simulink model "Bahnplanung_lauffaehig_auf_Robotino"  (R2015b)
settings: Solver=ode3  StartTime=0.0  StopTime=inf  FixedStep=0.005  RelTol=1e-3
undefined symbols (not defined in the file or in its folder): Com1, none
libraries: xpcobsoletelib x4, xpcrtudplib x3, simulink x2, xpcseriallib x1, slrtlib x1
(part 1 of 2)
CloseFcn:
  | rtwprivate ssgencode ModelCloseRequest Robotino_Strecke_reall_2009
settings Model: SimulationMode=external  Creator=atlabor  LastModifiedBy=atlabor
settings SolverCC: EnableConcurrentExecution=on
settings DataIOCC: LimitDataPoints=off  SaveFormat=Array  SignalLoggingSaveFormat=ModelDataLogs
settings OptimizationCC: BlockReduction=off  OptimizeBlockIOStorage=off  BufferReuse=off  GlobalBufferReuse=off  ExpressionFolding=off  ExpressionDepthLimit=2147483647  LocalBlockOutputs=off  InitFltsAndDblsToZero=on
settings DebuggingCC: SaveWithParameterizedLinksMsg=none  UnderspecifiedInitializationDetection=Classic  MergeDetectMultiDrivingBlocksExec=none  SolverPrmCheckMsg=warning  FcnCallInpInsideContextMsg=UseLocalSettings  StateNameClashWarn=warning
settings HardwareCC: ProdBitPerPointer=32  ProdLargestAtomicFloat=None  ProdWordSize=32  ProdLongLongMode=on  ProdHWDeviceType=Generic->32-bit x86 compatible
settings SFSimCC: SimParseCustomCode=off
settings RTWCC: SystemTargetFile=slrt.tlc  TemplateMakefile=slrt_default_tmf  Description=Simulink Real-Time  RTWCompilerOptimization=on
settings SimulinkRealTimeCC: GeneratePreprocessorConditionals=Disable all
settings ConfigComp: CovModelRefEnable=Off  CovSFcnEnable=off

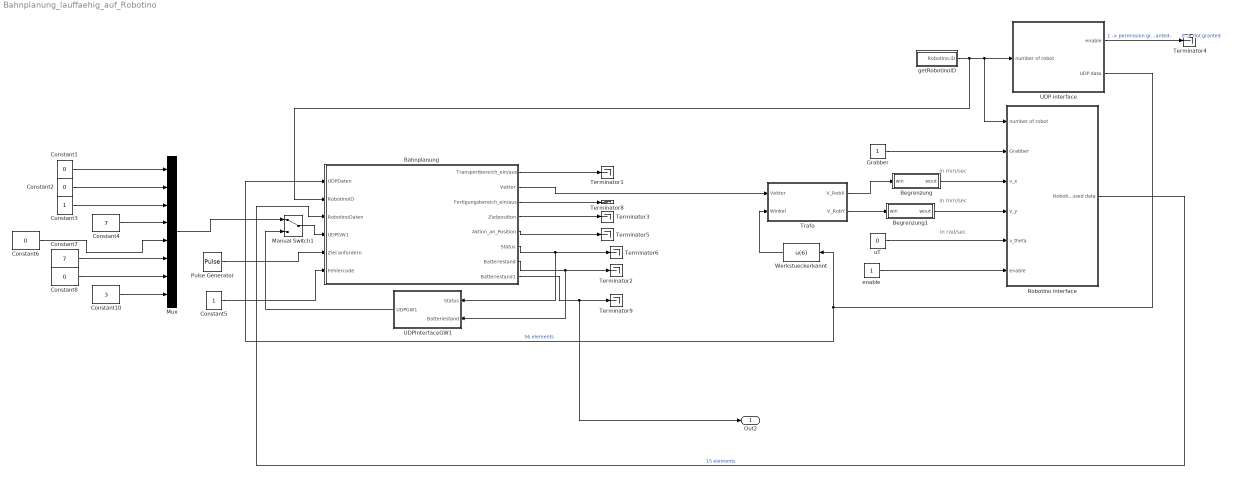
== system Bahnplanung_lauffaehig_auf_Robotino ==
  note: in rad/sec
  note: in mm/sec
  note: in mm/sec
  Bahnplanung : Subsystem
  Begrenzung : MATLAB Function  TreatAsAtomicUnit=on
  Begrenzung1 : MATLAB Function  TreatAsAtomicUnit=on
  Constant{1..2,6,8} (4 alike) : Constant  Value=0
  Constant10 : Constant  Value=3
  Constant3 : Constant
  Constant4 : Constant  Value=7
  Constant5 : Constant
  Constant7 : Constant  Value=7
  Grabber : Constant
  Manual Switch1 : ManualSwitch
  Mux : Mux  Inputs=8
  Pulse Generator : DiscretePulseGenerator  PulseType=Time based  Period=5  PulseWidth=50
  Robotino interface : Subsystem
  Terminator{1..6,8..9} (8 alike) : Terminator
  Trafo : MATLAB Function  TreatAsAtomicUnit=on
  UDP interface : Subsystem
  UDPInterfaceGW1 : Subsystem
  Werkstueckerkannt : Fcn  Expr=u(6)
  enable : Constant
  getRobotinoID : Subsystem
  uT : Constant  Value=0
  Out2 : Outport
  wires:
  Robotino interface/1(Robotino processed data) -> Bahnplanung/3(RobotinoDaten)  "15 elements"
  UDP interface/2(UDP data) -> Bahnplanung/1(UDPDaten), Werkstueckerkannt/1  "56 elements"
  uT/1 -> Robotino interface/5(v_theta)
  UDP interface/1(enable) -> Terminator4/1  "1 -> permission granted;        0 -> not granted"
  enable/1 -> Robotino interface/6(enable)
  getRobotinoID/1(Robotino.ID) -> Bahnplanung/2(RobotinoID), Robotino interface/1(number of robot), UDP interface/1(number of robot)
  Grabber/1 -> Robotino interface/2(Grabber)
  Constant5/1 -> Bahnplanung/6(Fehlercode)
  Pulse Generator/1 -> Bahnplanung/5(Ziel anfordern)
  Bahnplanung/1(Transportbereich_ein/aus) -> Terminator1/1
  Bahnplanung/4(Zielposition) -> Terminator3/1
  Bahnplanung/5(Aktion_an_Position) -> Terminator5/1
  Bahnplanung/6(Status) -> Terminator6/1, UDPInterfaceGW1/1(Status)
  Bahnplanung/7(Batteriestand) -> Terminator2/1, UDPInterfaceGW1/2(Batteriestand)
  Bahnplanung/3(Fertigungsbereich_ein/aus) -> Terminator8/1
  Constant1/1 -> Mux/1
  Constant2/1 -> Mux/2
  Constant3/1 -> Mux/3
  Constant6/1 -> Mux/5
  Constant7/1 -> Mux/6
  Constant8/1 -> Mux/7
  Constant10/1 -> Mux/8
  Begrenzung/1(wout) -> Robotino interface/3(v_x)
  Trafo/2(V_RobY) -> Begrenzung1/1(win)
  Werkstueckerkannt/1 -> Trafo/2(Winkel)
  Trafo/1(V_RobX) -> Begrenzung/1(win)
  Begrenzung1/1(wout) -> Robotino interface/4(v_y)
  Constant4/1 -> Mux/4
  Manual Switch1/1 -> Bahnplanung/4(UDPGW1)
  Mux/1 -> Manual Switch1/1
  UDPInterfaceGW1/1(UDPGW1) -> Manual Switch1/2
  Bahnplanung/8(Batteriestand1) -> Out2/1, Terminator9/1
  Bahnplanung/2(Vektor) -> Trafo/1(Vektor)

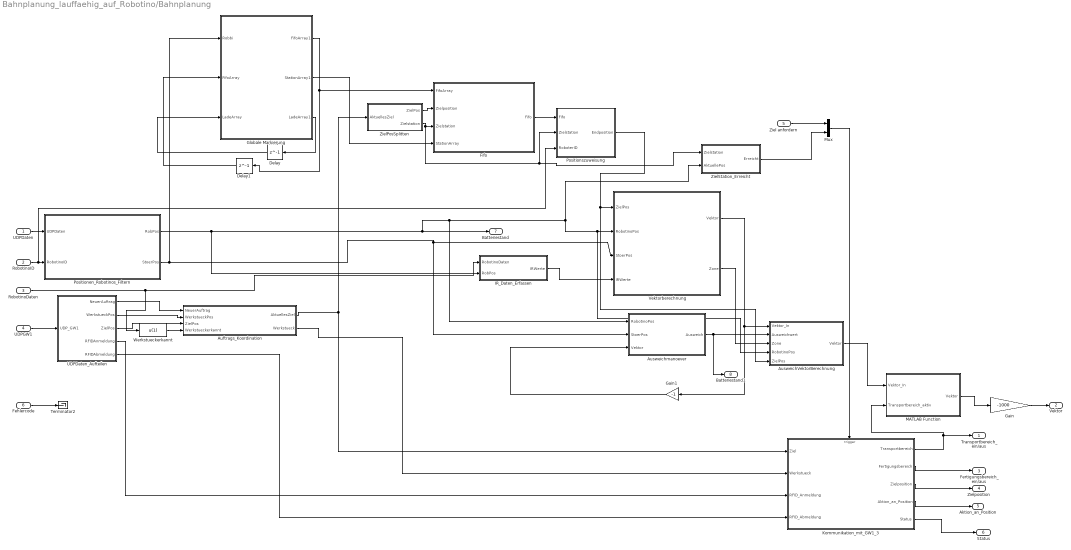
== system Bahnplanung_lauffaehig_auf_Robotino/Bahnplanung ==
  UDPDaten : Inport  PortDimensions=56
  RobotinoID : Inport  Port=2
  RobotinoDaten : Inport  Port=3
  UDPGW1 : Inport  Port=4
  Ziel anfordern : Inport  Port=5
  Fehlercode : Inport  Port=6
  Auftrags_Koordination : Stateflow chart  TreatAsAtomicUnit=on
  AusweichVektorBerechnung : MATLAB Function  TreatAsAtomicUnit=on
  Ausweichmanoever : MATLAB Function  TreatAsAtomicUnit=on
  Delay : Delay  DelayLength=1
  Delay1 : Delay  DelayLength=1
  Fifo : Stateflow chart  TreatAsAtomicUnit=on
  Gain : Gain  Gain=-1000
  Gain1 : Gain  Gain=-1
  Globale Markierung : MATLAB Function  TreatAsAtomicUnit=on
  IR_Daten_Erfassen : MATLAB Function  TreatAsAtomicUnit=on
  Kommunikation_mit_GW1_3 : Stateflow chart  TreatAsAtomicUnit=on
  MATLAB Function : MATLAB Function  TreatAsAtomicUnit=on
  Mux : Mux  Inputs=2
  Positionen_Robotinos_Filtern : MATLAB Function  TreatAsAtomicUnit=on
  Positionszuweisung : MATLAB Function  TreatAsAtomicUnit=on
  Terminator2 : Terminator
  UDPDaten_Aufteilen : Subsystem
  Vektorberechnung : MATLAB Function  TreatAsAtomicUnit=on
  Werkstueckerkannt : Fcn  Expr=u(1)
  ZielPosSplitten : MATLAB Function  TreatAsAtomicUnit=on
  ZielStation_Erreicht : MATLAB Function  TreatAsAtomicUnit=on
  Transportbereich_ein/aus : Outport
  Vektor : Outport  Port=2  OutDataTypeStr=double  PortDimensions=[1 2]
  Fertigungsbereich_ein/aus : Outport  Port=3
  Zielposition : Outport  Port=4
  Aktion_an_Position : Outport  Port=5
  Status : Outport  Port=6
  Batteriestand : Outport  Port=7
  Batteriestand1 : Outport  Port=8
  wires:
  RobotinoID/1 -> Positionszuweisung/3(RoboterID), Positionen_Robotinos_Filtern/2(RobotinoID)
  UDPDaten/1 -> Positionen_Robotinos_Filtern/1(UDPDaten)
  Positionen_Robotinos_Filtern/2(StoerPos) -> Ausweichmanoever/2(StoerPos), Vektorberechnung/3(StoerPos), Globale Markierung/1(Robbi)
  Globale Markierung/2(StationArray1) -> Fifo/4(StationArray)
  RobotinoDaten/1 -> IR_Daten_Erfassen/1(RobotinoDaten), Werkstueckerkannt/1
  Kommunikation_mit_GW1_3/3(Zielposition) -> Zielposition/1
  Kommunikation_mit_GW1_3/4(Aktion_an_Position) -> Aktion_an_Position/1
  Kommunikation_mit_GW1_3/2(Fertigungsbereich) -> Fertigungsbereich_ein/aus/1
  Kommunikation_mit_GW1_3/1(Transportbereich) -> Transportbereich_ein/aus/1, MATLAB Function/2(Transportbereich_aktiv)
  UDPGW1/1 -> UDPDaten_Aufteilen/1(UDP_GW1)
  UDPDaten_Aufteilen/4(RFIDAnmeldung) -> Kommunikation_mit_GW1_3/3(RFID_Anmeldung)
  UDPDaten_Aufteilen/5(RFIDAbmeldung) -> Kommunikation_mit_GW1_3/4(RFID_Abmeldung)
  UDPDaten_Aufteilen/2(WerkstueckPos) -> Auftrags_Koordination/2(WerkstueckPos)
  UDPDaten_Aufteilen/3(ZielPos) -> Auftrags_Koordination/3(ZielPos)
  Auftrags_Koordination/1(AktuellesZiel) -> ZielPosSplitten/1(AktuellesZiel), Kommunikation_mit_GW1_3/1(Ziel)
  ZielPosSplitten/1(ZielPos) -> Fifo/2(Zielposition)
  ZielPosSplitten/2(Zielstation) -> ZielStation_Erreicht/1(Zielstation), Positionszuweisung/2(Zielstation), Fifo/3(Zielstation)
  Fehlercode/1 -> Terminator2/1
  UDPDaten_Aufteilen/1(NeuerAuftrag) -> Auftrags_Koordination/1(NeuerAuftrag)
  Auftrags_Koordination/2(Werkstueck) -> Kommunikation_mit_GW1_3/2(Werkstueck)
  Werkstueckerkannt/1 -> Auftrags_Koordination/4(Werkstueckerkannt)
  Globale Markierung/1(FifoArray1) -> Delay1/1, Fifo/1(FifoArray)
  Delay1/1 -> Globale Markierung/2(FifoArray)
  Fifo/1(Fifo) -> Positionszuweisung/1(Fifo)
  Positionszuweisung/1(Endposition) -> AusweichVektorBerechnung/5(ZielPos), Vektorberechnung/1(ZielPos)
  Kommunikation_mit_GW1_3/5(Status) -> Status/1
  Globale Markierung/3(LadeArray1) -> Delay/1
  Delay/1 -> Globale Markierung/3(LadeArray)
  Mux/1 -> Kommunikation_mit_GW1_3/Trigger
  Ziel anfordern/1 -> Mux/1
  ZielStation_Erreicht/1(Erreicht) -> Mux/2
  MATLAB Function/1(Vektor) -> Gain/1
  Ausweichmanoever/1(Ausweich) -> Batteriestand1/1, AusweichVektorBerechnung/2(Ausweichwert)
  Gain/1 -> Vektor/1
  Vektorberechnung/1(Vektor) -> AusweichVektorBerechnung/1(Vektor_In), Gain1/1
  Gain1/1 -> Ausweichmanoever/3(Vektor)
  Positionen_Robotinos_Filtern/1(RobPos) -> IR_Daten_Erfassen/2(RobPos), Batteriestand/1, Ausweichmanoever/1(RobotinoPos), ZielStation_Erreicht/2(AktuellePos), AusweichVektorBerechnung/4(RobotinoPos), Vektorberechnung/2(RobotinoPos)
  IR_Daten_Erfassen/1(IRWerte) -> Vektorberechnung/4(IRWerte)
  AusweichVektorBerechnung/1(Vektor) -> MATLAB Function/1(Vektor_In)
  Vektorberechnung/2(Zone) -> AusweichVektorBerechnung/3(Zone)

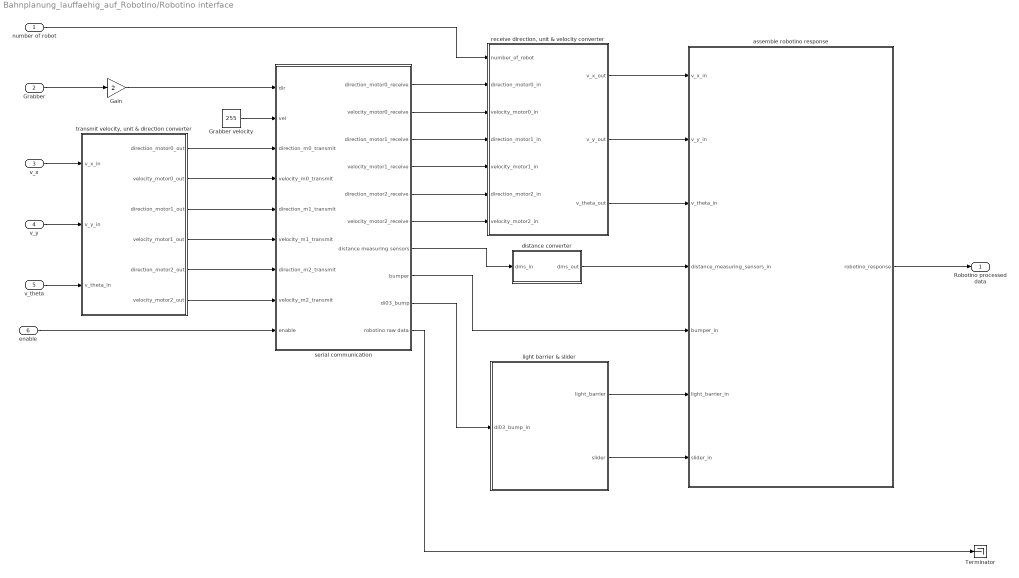
== system Bahnplanung_lauffaehig_auf_Robotino/Robotino interface ==
  number of robot : Inport
  Grabber : Inport  Port=2
  v_x : Inport  Port=3
  v_y : Inport  Port=4
  v_theta : Inport  Port=5
  enable : Inport  Port=6
  Gain : Gain  Gain=2
  Grabber velocity : Constant  Value=255
  Terminator : Terminator
  assemble robotino response : MATLAB Function  TreatAsAtomicUnit=on
  distance converter : MATLAB Function  TreatAsAtomicUnit=on
  light barrier & slider : MATLAB Function  TreatAsAtomicUnit=on
  "receive direction, unit & velocity converter" : MATLAB Function  TreatAsAtomicUnit=on
  serial communication : Subsystem
  "transmit velocity, unit & direction converter" : MATLAB Function  TreatAsAtomicUnit=on
  Robotino processed data : Outport
  wires:
  "transmit velocity, unit & direction converter"/1(direction_motor0_out) -> serial communication/3(direction_m0_transmit)
  "transmit velocity, unit & direction converter"/2(velocity_motor0_out) -> serial communication/4(velocity_m0_transmit)
  "transmit velocity, unit & direction converter"/3(direction_motor1_out) -> serial communication/5(direction_m1_transmit)
  "transmit velocity, unit & direction converter"/4(velocity_motor1_out) -> serial communication/6(velocity_m1_transmit)
  "transmit velocity, unit & direction converter"/5(direction_motor2_out) -> serial communication/7(direction_m2_transmit)
  "transmit velocity, unit & direction converter"/6(velocity_motor2_out) -> serial communication/8(velocity_m2_transmit)
  v_x/1 -> "transmit velocity, unit & direction converter"/1(v_x_in)
  v_y/1 -> "transmit velocity, unit & direction converter"/2(v_y_in)
  v_theta/1 -> "transmit velocity, unit & direction converter"/3(v_theta_in)
  "receive direction, unit & velocity converter"/2(v_y_out) -> assemble robotino response/2(v_y_in)
  enable/1 -> serial communication/9(enable)
  serial communication/1(direction_motor0_receive) -> "receive direction, unit & velocity converter"/2(direction_motor0_in)
  serial communication/7(distance measuring sensors) -> distance converter/1(dms_in)
  serial communication/10(robotino raw data) -> Terminator/1
  serial communication/9(di03_bump) -> light barrier & slider/1(di03_bump_in)
  "receive direction, unit & velocity converter"/1(v_x_out) -> assemble robotino response/1(v_x_in)
  "receive direction, unit & velocity converter"/3(v_theta_out) -> assemble robotino response/3(v_theta_in)
  assemble robotino response/1(robotino_response) -> Robotino processed data/1
  Grabber/1 -> Gain/1
  Gain/1 -> serial communication/1(dir)
  distance converter/1(dms_out) -> assemble robotino response/4(distance_measuring_sensors_in)
  light barrier & slider/2(slider) -> assemble robotino response/7(slider_in)
  light barrier & slider/1(light_barrier) -> assemble robotino response/6(light_barrier_in)
  serial communication/8(bumper) -> assemble robotino response/5(bumper_in)
  serial communication/2(velocity_motor0_receive) -> "receive direction, unit & velocity converter"/3(velocity_motor0_in)
  serial communication/3(direction_motor1_receive) -> "receive direction, unit & velocity converter"/4(direction_motor1_in)
  serial communication/4(velocity_motor1_receive) -> "receive direction, unit & velocity converter"/5(velocity_motor1_in)
  serial communication/5(direction_motor2_receive) -> "receive direction, unit & velocity converter"/6(direction_motor2_in)
  serial communication/6(velocity_motor2_receive) -> "receive direction, unit & velocity converter"/7(velocity_motor2_in)
  Grabber velocity/1 -> serial communication/2(vel)
  number of robot/1 -> "receive direction, unit & velocity converter"/1(number_of_robot)

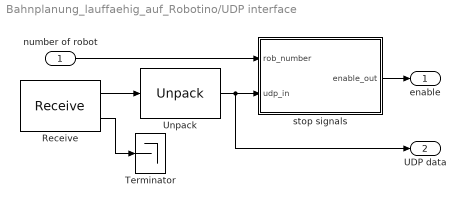
== system Bahnplanung_lauffaehig_auf_Robotino/UDP interface ==
  number of robot : Inport
  Receive : xpcrtudplib/Legacy UDP/Receive   ipAddress=0.0.0.0  ipPort=25000  width=448  vblLen=off  sampletime=-1
  Terminator : Terminator
  Unpack : xpcobsoletelib/Utilities/Unpack   dimensions={[56]}  datatypes={'double'}  byteAlign=1
  stop signals : MATLAB Function  TreatAsAtomicUnit=on
  enable : Outport
  UDP data : Outport  Port=2
  wires:
  Unpack/1 -> stop signals/2(udp_in), UDP data/1
  Receive/1 -> Unpack/1
  Receive/2 -> Terminator/1
  stop signals/1(enable_out) -> enable/1
  number of robot/1 -> stop signals/1(rob_number)

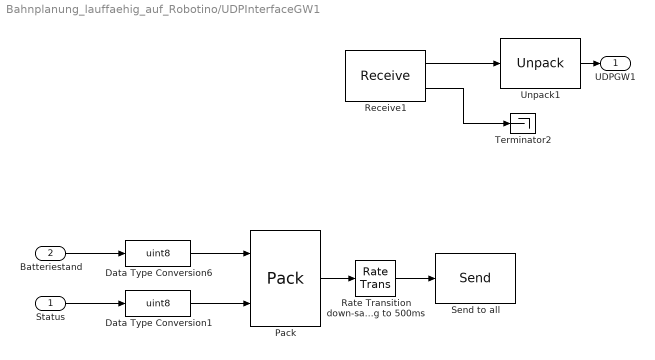
== system Bahnplanung_lauffaehig_auf_Robotino/UDPInterfaceGW1 ==
  Status : Inport
  Batteriestand : Inport  Port=2
  Data Type Conversion1 : DataTypeConversion  OutDataTypeStr=uint8
  Data Type Conversion6 : DataTypeConversion  OutDataTypeStr=uint8
  Pack : xpcobsoletelib/Utilities/Pack   datatypes={'int16','int16'}  byteAlign=1
  Rate Transition down-sampling to 500ms : RateTransition  OutPortSampleTime=0.5
  Receive1 : xpcrtudplib/Legacy UDP/Receive   ipAddress=0.0.0.0  ipPort=20000  width=448  vblLen=off  sampletime=-1
  Send to all : xpcrtudplib/Legacy UDP/Send   ipAddress=255.255.255.255  ipPort=20000  localPort=-1  vblLen=off  sampletime=-1
  Terminator2 : Terminator
  Unpack1 : xpcobsoletelib/Utilities/Unpack   dimensions={[8]}  datatypes={'int8'}  byteAlign=1
  UDPGW1 : Outport
  wires:
  Receive1/2 -> Terminator2/1
  Unpack1/1 -> UDPGW1/1
  Receive1/1 -> Unpack1/1
  Pack/1 -> Rate Transition down-sampling to 500ms/1
  Rate Transition down-sampling to 500ms/1 -> Send to all/1
  Data Type Conversion1/1 -> Pack/2
  Data Type Conversion6/1 -> Pack/1
  Batteriestand/1 -> Data Type Conversion6/1
  Status/1 -> Data Type Conversion1/1

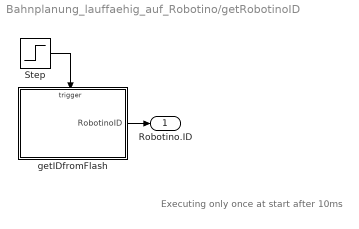
== system Bahnplanung_lauffaehig_auf_Robotino/getRobotinoID ==
  note: Executing only once at start after 10ms
  Step : Step  Time=0.01  SampleTime=0
  getIDfromFlash : Subsystem
  Robotino.ID : Outport
  wires:
  Step/1 -> getIDfromFlash/Trigger
  getIDfromFlash/1(RobotinoID) -> Robotino.ID/1

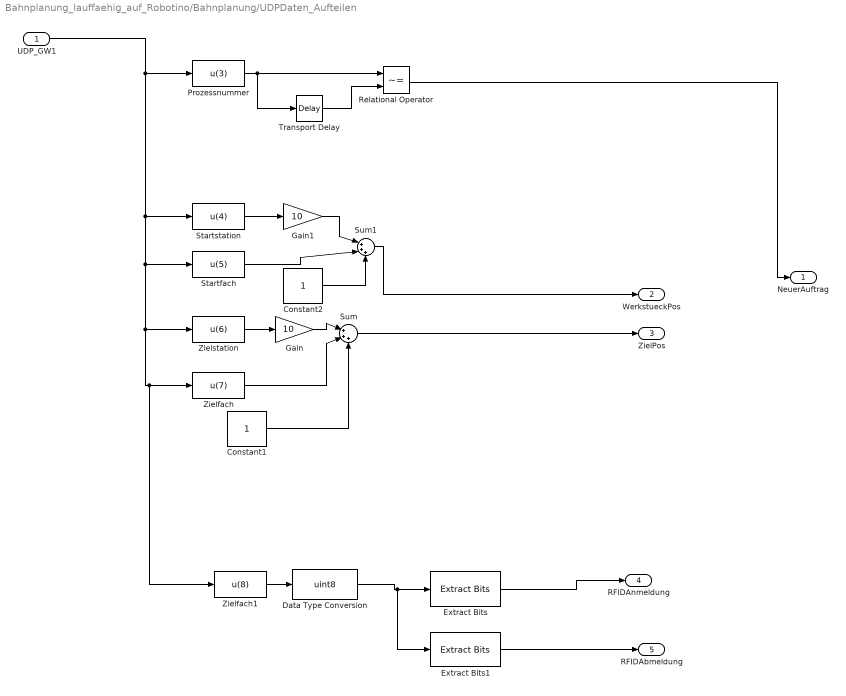
== system Bahnplanung_lauffaehig_auf_Robotino/Bahnplanung/UDPDaten_Aufteilen ==
  UDP_GW1 : Inport
  Constant1 : Constant
  Constant2 : Constant
  Data Type Conversion : DataTypeConversion  OutDataTypeStr=uint8
  Extract Bits : simulink/Logic and Bit Operations/Extract Bits  bitsToExtract=Range of bits  numBits=8  bitIdxRange=[0]  outScalingMode=Treat bit field as an integer
  Extract Bits1 : simulink/Logic and Bit Operations/Extract Bits  bitsToExtract=Range of bits  numBits=8  bitIdxRange=[1]  outScalingMode=Treat bit field as an integer
  Gain : Gain  Gain=10
  Gain1 : Gain  Gain=10
  Prozessnummer : Fcn  Expr=u(3)
  Relational Operator : RelationalOperator  Operator=~=  OutDataTypeStr=boolean
  Startfach : Fcn  Expr=u(5)
  Startstation : Fcn  Expr=u(4)
  Sum : Sum  Inputs=|+++
  Sum1 : Sum  Inputs=|+++
  Transport Delay : TransportDelay
  Zielfach : Fcn  Expr=u(7)
  Zielfach1 : Fcn  Expr=u(8)
  Zielstation : Fcn  Expr=u(6)
  NeuerAuftrag : Outport
  WerkstueckPos : Outport  Port=2
  ZielPos : Outport  Port=3
  RFIDAnmeldung : Outport  Port=4
  RFIDAbmeldung : Outport  Port=5
  wires:
  Zielfach/1 -> Sum/2
  Gain/1 -> Sum/1
  Zielstation/1 -> Gain/1
  UDP_GW1/1 -> Prozessnummer/1, Zielfach1/1, Zielfach/1, Zielstation/1, Startfach/1, Startstation/1
  Sum1/1 -> WerkstueckPos/1
  Startfach/1 -> Sum1/2
  Gain1/1 -> Sum1/1
  Constant2/1 -> Sum1/3
  Startstation/1 -> Gain1/1
  Constant1/1 -> Sum/3
  Sum/1 -> ZielPos/1
  Relational Operator/1 -> NeuerAuftrag/1
  Zielfach1/1 -> Data Type Conversion/1
  Data Type Conversion/1 -> Extract Bits1/1, Extract Bits/1
  Prozessnummer/1 -> Transport Delay/1, Relational Operator/1
  Transport Delay/1 -> Relational Operator/2
  Extract Bits1/1 -> RFIDAbmeldung/1
  Extract Bits/1 -> RFIDAnmeldung/1

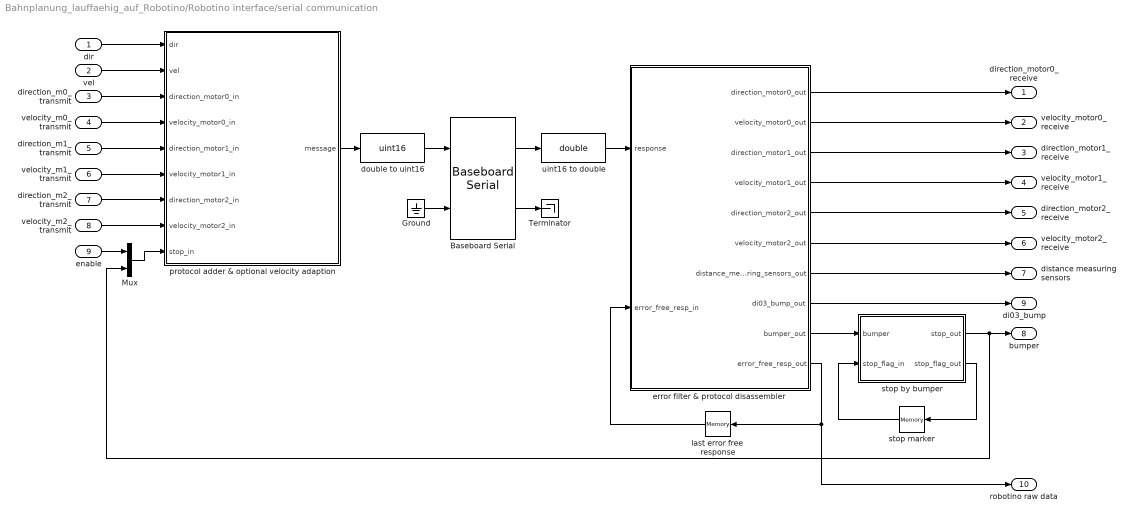
== system Bahnplanung_lauffaehig_auf_Robotino/Robotino interface/serial communication ==
  dir : Inport
  vel : Inport  Port=2
  direction_m0_transmit : Inport  Port=3
  velocity_m0_transmit : Inport  Port=4
  direction_m1_transmit : Inport  Port=5
  velocity_m1_transmit : Inport  Port=6
  direction_m2_transmit : Inport  Port=7
  velocity_m2_transmit : Inport  Port=8
  enable : Inport  Port=9
  Baseboard Serial : xpcseriallib/Mainboard/Baseboard Serial  group=Transmit Setup  port=2  irqnum=4  saddr1=0x3f8  saddr2=0x3e8  config=Com1/none  baud1=115200  parity1=None  ndata1=8  nstop1=1  fifomode1=16 deep  rlevel1=almost full  automode1=off  xmtfifosize1=10240  xmtdatatype1=count+16 bit uint  rcvfifosize1=10240  rcvmaxread1=101  rcvminread1=1  rcvusedelim1=on  rcvdelim1=99  rcvdatatype1=count+16 bit uint  rcvsampletime1=-1  baud2=115200  parity2=None  ndata2=8  nstop2=1  fifomode2=16 deep  rlevel2=almost full  automode2=off  xmtfifosize2=10240  xmtdatatype2=count+16 bit uint  rcvfifosize2=10240  rcvmaxread2=101  rcvminread2=1  rcvusedelim2=on  rcvdelim2=99  rcvdatatype2=count+16 bit uint  rcvsampletime2=-1
      link override FIFO read 1: maxsize=101  minsize=1  usedelimiter=on  delimiter=99  outputtype=count+16 bit uint  sampletime=dt / 2
      link override FIFO read 2: maxsize=101  minsize=1  usedelimiter=on  delimiter=99  outputtype=count+16 bit uint  sampletime=dt / 2
      link override FIFO write 1: size=1024  inputtype=count+16 bit uint  sampletime=-1  id=XMT channel 1, IRQ 4
      link override FIFO write 2: size=1024  inputtype=8 bit uint null terminated  id=XMT channel 2, IRQ 4
      link override Setup1: baud=115200  width=8  nstop=1  parity=None  fmode=16 deep  rlevel=half full  ctsmode=off
      link override Setup2: baud=4800  width=8  nstop=1  parity=None  fmode=16 deep  rlevel=half full  ctsmode=off
  Ground : Ground
  Mux : Mux  Inputs=2
  Terminator : Terminator
  double to uint16 : DataTypeConversion  OutDataTypeStr=uint16  RndMeth=Nearest
  error filter & protocol disassembler : MATLAB Function  TreatAsAtomicUnit=on
  last error free response : Memory  X0=[zeros(1,102)]
  protocol adder & optional velocity adaption : MATLAB Function  TreatAsAtomicUnit=on
  stop by bumper : MATLAB Function  TreatAsAtomicUnit=on
  stop marker : Memory  X0=[zeros(1,3)]
  uint16 to double : DataTypeConversion  OutDataTypeStr=double  RndMeth=Nearest
  direction_motor0_receive : Outport
  velocity_motor0_receive : Outport  Port=2
  direction_motor1_receive : Outport  Port=3
  velocity_motor1_receive : Outport  Port=4
  direction_motor2_receive : Outport  Port=5
  velocity_motor2_receive : Outport  Port=6
  distance measuring sensors : Outport  Port=7
  bumper : Outport  Port=8
  di03_bump : Outport  Port=9
  robotino raw data : Outport  Port=10
  wires:
  Ground/1 -> Baseboard Serial/2
  Baseboard Serial/2 -> Terminator/1
  double to uint16/1 -> Baseboard Serial/1
  protocol adder & optional velocity adaption/1(message) -> double to uint16/1
  stop marker/1 -> stop by bumper/2(stop_flag_in)
  stop by bumper/2(stop_flag_out) -> stop marker/1
  last error free response/1 -> error filter & protocol disassembler/2(error_free_resp_in)
  error filter & protocol disassembler/10(error_free_resp_out) -> last error free response/1, robotino raw data/1
  error filter & protocol disassembler/1(direction_motor0_out) -> direction_motor0_receive/1
  error filter & protocol disassembler/2(velocity_motor0_out) -> velocity_motor0_receive/1
  error filter & protocol disassembler/3(direction_motor1_out) -> direction_motor1_receive/1
  error filter & protocol disassembler/4(velocity_motor1_out) -> velocity_motor1_receive/1
  direction_m0_transmit/1 -> protocol adder & optional velocity adaption/3(direction_motor0_in)
  error filter & protocol disassembler/5(direction_motor2_out) -> direction_motor2_receive/1
  velocity_m0_transmit/1 -> protocol adder & optional velocity adaption/4(velocity_motor0_in)
  error filter & protocol disassembler/6(velocity_motor2_out) -> velocity_motor2_receive/1
  direction_m1_transmit/1 -> protocol adder & optional velocity adaption/5(direction_motor1_in)
  velocity_m1_transmit/1 -> protocol adder & optional velocity adaption/6(velocity_motor1_in)
  direction_m2_transmit/1 -> protocol adder & optional velocity adaption/7(direction_motor2_in)
  velocity_m2_transmit/1 -> protocol adder & optional velocity adaption/8(velocity_motor2_in)
  error filter & protocol disassembler/9(bumper_out) -> stop by bumper/1(bumper)
  stop by bumper/1(stop_out) -> bumper/1, Mux/2
  error filter & protocol disassembler/7(distance_measuring_sensors_out) -> distance measuring sensors/1
  Baseboard Serial/1 -> uint16 to double/1
  uint16 to double/1 -> error filter & protocol disassembler/1(response)
  enable/1 -> Mux/1
  dir/1 -> protocol adder & optional velocity adaption/1(dir)
  vel/1 -> protocol adder & optional velocity adaption/2(vel)
  Mux/1 -> protocol adder & optional velocity adaption/9(stop_in)
  error filter & protocol disassembler/8(di03_bump_out) -> di03_bump/1

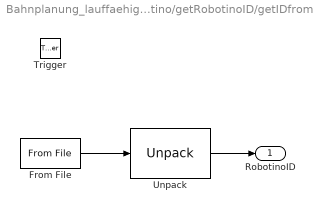
== system Bahnplanung_lauffaehig_auf_Robotino/getRobotinoID/getIDfromFlash ==
  Trigger : TriggerPort
  From File : slrtlib/Target Management/From File   filename='robotino.id'  dataSize=8  bufSize=2000  readSize=512  EOFOption=Seek to beginning  sampTime=-1  show2ports=off
  Unpack : xpcobsoletelib/Utilities/Unpack   dimensions={[1]}  datatypes={'double'}  byteAlign=1
  RobotinoID : Outport
  wires:
  From File/1 -> Unpack/1
  Unpack/1 -> RobotinoID/1

== matlab function Bahnplanung_lauffaehig_auf_Robotino/Robotino interface/transmit velocity, unit & direction converter ==
  settings: sampleTime=2*dtpc
  data: direction_motor0_out output; velocity_motor0_out output; direction_motor1_out output; velocity_motor1_out output; direction_motor2_out output; velocity_motor2_out output; v_x_in input; v_y_in input; v_theta_in input
%%%%%%%%%%%%%%%%%%%%%%%%%%%%%%%%%%%%%%%%%%%%%%%%%%%%%%%%%%%%%%%%%%%%%%%%%%%
% conversion from positive and/or negative longitudinal, lateral and      %
% rotational velocities (in milimeters per second) to three separate      %
% positive motor velocities (resolution: 1Byte) and their rotation        %
% direction                                                               %
%                                                                         %
% inputs:  v_x_in (longitudinal velocity in milimeters per second),       %
%          v_y_in (lateral velocity in milimeters per second),            %
%          v_theta_in (rotational velocity in milimeters per second)      %
% outputs: direction_motor0_out (rotating direction of motor0             %
%          (0 := counter-clockwise; 2 := clockwise)),                     %
%          velocity_motor0_out (from 0 to 255),                           %
%          direction_motor1_out (rotating direction of motor1             %
%          (0 := counter-clockwise; 2 := clockwise)),                     %
%          velocity_motor1_out (from 0 to 255),                           %
%          direction_motor2_out (rotating direction of motor2             %
%          (0 := counter-clockwise; 2 := clockwise)),                     %
%          velocity_motor2_out (from 0 to 255)                            %
%%%%%%%%%%%%%%%%%%%%%%%%%%%%%%%%%%%%%%%%%%%%%%%%%%%%%%%%%%%%%%%%%%%%%%%%%%%
function [direction_motor0_out, velocity_motor0_out, ...
          direction_motor1_out, velocity_motor1_out, ...
          direction_motor2_out, velocity_motor2_out] ...
                                          = fcn(v_x_in, v_y_in, v_theta_in)
%%%%%%%%%%%%%%%%%%%%%%%%%%%%%%%%%%%%%%%%%%%%%%%%%%%%%%%%%%%%%%%%%%%%%%
% conversion from longitudinal, lateral & rotational velocity to the %
% three separate motor velocities                                    %
%%%%%%%%%%%%%%%%%%%%%%%%%%%%%%%%%%%%%%%%%%%%%%%%%%%%%%%%%%%%%%%%%%%%%%
v0 = (-v_x_in * cosd(30)) + ( v_y_in * cosd(60)) + (v_theta_in * 135);
v1 =                      + (-v_y_in)            + (v_theta_in * 135);
v2 = ( v_x_in * cosd(30)) + ( v_y_in * cosd(60)) + (v_theta_in * 135);

%%%%%%%%%%%%%%%%%%%%%%%%%%%%%%%%%%%%%%%%%%%%%%%%%%%%%%%%%%%%%%%%%%%%%
% conversion of the separate motor velocities from millimeters to a %
% value between -255 and 255                                        %
%%%%%%%%%%%%%%%%%%%%%%%%%%%%%%%%%%%%%%%%%%%%%%%%%%%%%%%%%%%%%%%%%%%%%
f = 1 / 7.02;
v0 = v0 * f;
v1 = v1 * f;
v2 = v2 * f;

%%%%%%%%%%%%%%%%%%%%%%%%%%%%%%%%%%%%%%%%%%%%%%%%%%%%%%%%%%%%%%%%%%%%
% division of motor velocities into absolute velocity and rotating %
% direction                                                        %
%%%%%%%%%%%%%%%%%%%%%%%%%%%%%%%%%%%%%%%%%%%%%%%%%%%%%%%%%%%%%%%%%%%%
if v0 < 0
    direction_motor0_out =  0;
    velocity_motor0_out  = -v0;
else
    direction_motor0_out = 2;
    velocity_motor0_out  = v0;
end

if v1 < 0
    direction_motor1_out =  0;
    velocity_motor1_out  = -v1;
else
    direction_motor1_out = 2;
    velocity_motor1_out  = v1;
end

if v2 < 0
    direction_motor2_out =  0;
    velocity_motor2_out  = -v2;
else
    direction_motor2_out = 2;
    velocity_motor2_out  = v2;
end

== matlab function Bahnplanung_lauffaehig_auf_Robotino/Robotino interface/serial communication/protocol adder & optional velocity adaption ==
  settings: sampleTime=2*dtpc
  data: dir input; vel input; direction_motor0_in input; velocity_motor0_in input; direction_motor1_in input; velocity_motor1_in input; direction_motor2_in input; velocity_motor2_in input; stop_in input; message output
%%%%%%%%%%%%%%%%%%%%%%%%%%%%%%%%%%%%%%%%%%%%%%%%%%%%%%%%%%%%%%%%%%%%%%%%%%%
% parameterising the 'PC104 to I/O-Board message' for serial line         %
% communication with control commands for the robotino motors             %
%                                                                         %
% optional: velocity adaption as soon as at least one motor is near the   %
%           speed limit                                                   %
%                                                                         %
% inputs: rotating directions and velocities of the three motors          %
% output: vector containing the 'PC104 to I/O-Board message' for serial   %
%         line communication                                              %
%%%%%%%%%%%%%%%%%%%%%%%%%%%%%%%%%%%%%%%%%%%%%%%%%%%%%%%%%%%%%%%%%%%%%%%%%%%
function message = fcn(dir, vel, direction_motor0_in, velocity_motor0_in, ...
                       direction_motor1_in, velocity_motor1_in, ...
                       direction_motor2_in, velocity_motor2_in, stop_in)
%%%%%%%%%%%%%%%%%%%%%%%%%%%%%%
% optional velocity adaption %
%%%%%%%%%%%%%%%%%%%%%%%%%%%%%%
vmax = 175;                                               % v_motor_dez_max

if velocity_motor0_in > vmax
    velocity_motor0_tf = velocity_motor0_in;
    
    velocity_motor0_in = vmax;
    velocity_motor1_in = vmax * velocity_motor1_in / velocity_motor0_tf;
    velocity_motor2_in = vmax * velocity_motor2_in / velocity_motor0_tf;
end

if velocity_motor1_in > vmax
    velocity_motor1_tf = velocity_motor1_in;
    
    velocity_motor0_in = vmax * velocity_motor0_in / velocity_motor1_tf;
    velocity_motor1_in = vmax;
    velocity_motor2_in = vmax * velocity_motor2_in / velocity_motor1_tf;
end

if velocity_motor2_in > vmax
    velocity_motor2_tf = velocity_motor2_in;
    
    velocity_motor0_in = vmax * velocity_motor0_in / velocity_motor2_tf;
    velocity_motor1_in = vmax * velocity_motor1_in / velocity_motor2_tf;
    velocity_motor2_in = vmax;
end
%%%%%%%%%%%%%%%%%%%%%%%%%%%%%%%%%%%%%%%%%%%%%%%%%%%%%%%%%%%%%%%%%%%%%%
% vector containing the 'PC104 to I/O-Board message' for serial line %
% communication                                                      %
%%%%%%%%%%%%%%%%%%%%%%%%%%%%%%%%%%%%%%%%%%%%%%%%%%%%%%%%%%%%%%%%%%%%%%
message = [47, abs('REC'), 5, min(stop_in), direction_motor0_in, ...
           velocity_motor0_in, zeros(1, 4), 255, 255, 255, ...
           min(stop_in), direction_motor1_in, velocity_motor1_in, ...
           zeros(1, 4), 255, 255, 255, min(stop_in), ...
           direction_motor2_in, velocity_motor2_in, zeros(1, 4), 255, ...
           255, 255, 1, dir, vel, zeros(1, 4), 255, 255, 255, abs('rec')].';

== matlab function Bahnplanung_lauffaehig_auf_Robotino/UDP interface/stop signals ==
  data: rob_number input; udp_in input; enable_out output
%%%%%%%%%%%%%%%%%%%%%%%%%%%%%%%%%%%%%%%%%%%%%%%%%%%%%%%%%%%%%%%%%%%%%%%%%%%
% Leads the enable command through. The enable command turns the Robotino %
% inputs to selectable form.                                              %
%                                                                         %
% input: udp_in (vector of 56 elements containing the data sent by the    %
%                camera-model)                                            %
% outputs: enable_out (1 = inputs are in selectable form;                 %
%                      0 = inputs are set to 0)                           %
%          udp_out (vector of 56 elements containing the data sent by the %
%                   camera-model)                                         %
%%%%%%%%%%%%%%%%%%%%%%%%%%%%%%%%%%%%%%%%%%%%%%%%%%%%%%%%%%%%%%%%%%%%%%%%%%%
function enable_out  = fcn(rob_number, udp_in)
enable_out = [0, 0];
if (udp_in(rob_number * 3 - 2) <= 0) && ...
   (udp_in(rob_number * 3 - 1) <= 0) && (udp_in(rob_number * 3) <= 0)
    enable_out(1) = 0;
else
    enable_out(1) = 1;
end
enable_out(2) = udp_in(28);

== matlab function Bahnplanung_lauffaehig_auf_Robotino/Robotino interface/serial communication/error filter & protocol disassembler ==
  settings: sampleTime=dtpc/2
  data: response input; error_free_resp_in input; direction_motor0_out output; velocity_motor0_out output; direction_motor1_out output; velocity_motor1_out output; direction_motor2_out output; velocity_motor2_out output; distance_measuring_sensors_out output; di03_bump_out output; bumper_out output; error_free_resp_out output
%%%%%%%%%%%%%%%%%%%%%%%%%%%%%%%%%%%%%%%%%%%%%%%%%%%%%%%%%%%%%%%%%%%%%%%%%%%
% Error check of the 'I/O-Board to PC104 message' and filtering of this   %
% defective response: Substitute defective message by the last error free %
% message.                                                                %
% Saving of the rotating direction, velocity, shaft position and running  %
% time of the three motors. Combining all shaft positions in a vector.    %
% Combining all running times in a vector.                                %
% Saving of the three bumper bytes indicating a collision in a vector.    %
% Saving the values of the nine distance measuring IR-sensors in a vector.%
%                                                                         %
% inputs: response (actual 'I/O-Board to PC104 message')(vector 102       %
%                   elements)                                             %
%         error_free_resp_in (last error free 'I/O-Board to PC104         %
%                             message')                                   %
% outputs: directions and velocities of the three motors                  %
%          motor_positions_out (shaft positions of the three motors)      %
%                              (vector 12 elements)                       %
%          time_bytes_out (running times of the three motors)             %
%                         (vector 9 elements)                             %
%          distance_measuring_sensors_out (values of the nine IR-sensors) %
%                                         (vector 9 elements)             %
%          bumper_out (vector 3 elements)                                 %
%          error_free_resp_out (error free 'I/O-Board to PC104 message')  %
%                              (vector 102 elements)                      %
%%%%%%%%%%%%%%%%%%%%%%%%%%%%%%%%%%%%%%%%%%%%%%%%%%%%%%%%%%%%%%%%%%%%%%%%%%%
function [direction_motor0_out, velocity_motor0_out, ...
          direction_motor1_out, velocity_motor1_out, ...
          direction_motor2_out, velocity_motor2_out, ...
          distance_measuring_sensors_out, di03_bump_out, bumper_out, ...
          error_free_resp_out] = fcn(response, error_free_resp_in)
%           motor_positions_out, time_bytes_out, ...)
      
%%%%%%%%%%%%%%%%%%%%%%%%%%%%%%%%%%%%%%%%%%%%%%%%%%%%%
% filtering defective 'I/O-Board to PC104 messages' %
%%%%%%%%%%%%%%%%%%%%%%%%%%%%%%%%%%%%%%%%%%%%%%%%%%%%%
if (response(1) == 101) && (response(2) == 82) && (response(3) == 69) ...
   && (response(4) == 67) && (response(100) == 114) ...        % if the ...
   && (response(101) == 101) && (response(102) == 99)  % counter (101), ...
                        % the start (REC) and stop (rec) bytes are true ...
    error_free_resp_out = response;     % save the actual 'I/O-Board to ...
                                                           % PC104 message'
else                                                        % otherwise ...
    error_free_resp_out = error_free_resp_in;     % save the last error ...
                                        % free 'I/O-Board to PC104 message'
end

%%%%%%%%%%%%%%%%%%%%%%%%%%%%%%%%%%%%%%%%%%%%%%%%%%%%%%%%%%%%%%%%%%%%%%%%%%
% save rotating direction, velocity, shaft position and the running time %
% of motor0                                                              %
%%%%%%%%%%%%%%%%%%%%%%%%%%%%%%%%%%%%%%%%%%%%%%%%%%%%%%%%%%%%%%%%%%%%%%%%%%
direction_motor0_out  = error_free_resp_out(26);
velocity_motor0_out   = error_free_resp_out(27);
% position_motor0_byte1 = error_free_resp_out(28);
% position_motor0_byte2 = error_free_resp_out(29);
% position_motor0_byte3 = error_free_resp_out(30);
% position_motor0_byte4 = error_free_resp_out(31);
% time_motor0_byte1     = error_free_resp_out(34);
% time_motor0_byte2     = error_free_resp_out(35);
% time_motor0_byte3     = error_free_resp_out(36);

%%%%%%%%%%%%%%%%%%%%%%%%%%%%%%%%%%%%%%%%%%%%%%%%%%%%%%%%%%%%%%%%%%%%%%%%%%
% save rotating direction, velocity, shaft position and the running time %
% of motor1                                                              %
%%%%%%%%%%%%%%%%%%%%%%%%%%%%%%%%%%%%%%%%%%%%%%%%%%%%%%%%%%%%%%%%%%%%%%%%%%
direction_motor1_out  = error_free_resp_out(47);
velocity_motor1_out   = error_free_resp_out(48);
% position_motor1_byte1 = error_free_resp_out(49);
% position_motor1_byte2 = error_free_resp_out(50);
% position_motor1_byte3 = error_free_resp_out(51);
% position_motor1_byte4 = error_free_resp_out(52);
% time_motor1_byte1     = error_free_resp_out(55);
% time_motor1_byte2     = error_free_resp_out(56);
% time_motor1_byte3     = error_free_resp_out(57);

%%%%%%%%%%%%%%%%%%%%%%%%%%%%%%%%%%%%%%%%%%%%%%%%%%%%%%%%%%%%%%%%%%%%%%%%%%
% save rotating direction, velocity, shaft position and the running time %
% of motor2                                                              %
%%%%%%%%%%%%%%%%%%%%%%%%%%%%%%%%%%%%%%%%%%%%%%%%%%%%%%%%%%%%%%%%%%%%%%%%%%
direction_motor2_out  = error_free_resp_out(68);
velocity_motor2_out   = error_free_resp_out(69);
% position_motor2_byte1 = error_free_resp_out(70);
% position_motor2_byte2 = error_free_resp_out(71);
% position_motor2_byte3 = error_free_resp_out(72);
% position_motor2_byte4 = error_free_resp_out(73);
% time_motor2_byte1     = error_free_resp_out(76);
% time_motor2_byte2     = error_free_resp_out(77);
% time_motor2_byte3     = error_free_resp_out(78);

%%%%%%%%%%%%%%%%%%%%%%%%%%%%%%%%%%%%%%%%%%%
% save the three bumper bytes in a vector %
%%%%%%%%%%%%%%%%%%%%%%%%%%%%%%%%%%%%%%%%%%%
bumper_out = [error_free_resp_out(32), error_free_resp_out(53), ...
              error_free_resp_out(74)]';
          
%%%%%%%%%%%%%%%%%%%%%%%%%%%%%%%%%%%%%%%%%%%%%%%%%%%%%%%%%%%%%%%%%%%%%%
% save the values of the nine distance measuring sensors in a vector %
%%%%%%%%%%%%%%%%%%%%%%%%%%%%%%%%%%%%%%%%%%%%%%%%%%%%%%%%%%%%%%%%%%%%%%
distance_measuring_sensors_out = [error_free_resp_out(60), ...
                    error_free_resp_out(59), error_free_resp_out(44), ...
                    error_free_resp_out(39), error_free_resp_out(38), ...
                    error_free_resp_out(17), error_free_resp_out(18), ...
                    error_free_resp_out(23), error_free_resp_out(65)];
                
%%%%%%%%%%%%%%%%%%%%%%%%%%%%%%%%%%%%%%%%%%%%%%%%%%%%%%%%
% save positions of the three motor shafts in a vector %
%%%%%%%%%%%%%%%%%%%%%%%%%%%%%%%%%%%%%%%%%%%%%%%%%%%%%%%%
% motor_positions_out = [position_motor0_byte1, position_motor0_byte2, ...
%                        position_motor0_byte3, position_motor0_byte4, ...
%                        position_motor1_byte1, position_motor1_byte2, ...
%                        position_motor1_byte3, position_motor1_byte4, ...
%                        position_motor2_byte1, position_motor2_byte2, ...
%                        position_motor2_byte3, position_motor2_byte4];

%%%%%%%%%%%%%%%%%%%%%%%%%%%%%%%%%%%%%%%%%%%%%%%%%%%%%%%%%%
% save the running times of the three motors in a vector %
%%%%%%%%%%%%%%%%%%%%%%%%%%%%%%%%%%%%%%%%%%%%%%%%%%%%%%%%%%
% time_bytes_out = [time_motor0_byte1, time_motor0_byte2, ...
%                   time_motor0_byte3, time_motor1_byte1, ...
%                   time_motor1_byte2, time_motor1_byte3, ...
%                   time_motor2_byte1, time_motor2_byte2, time_motor2_byte3];

%%%%%%%%%%%%%%%%%%%%%%%%%%%%%%%%%%%%%%
% save values of digital input 0 - 3 %
%%%%%%%%%%%%%%%%%%%%%%%%%%%%%%%%%%%%%%
di03_bump_out = error_free_resp_out(32);

== matlab function Bahnplanung_lauffaehig_auf_Robotino/Robotino interface/receive direction, unit & velocity converter ==
  settings: sampleTime=dtpc/2
  data: number_of_robot input; direction_motor0_in input; v_x_out output; velocity_motor0_in input; direction_motor1_in input; velocity_motor1_in input; direction_motor2_in input; velocity_motor2_in input; v_y_out output; v_theta_out output
%%%%%%%%%%%%%%%%%%%%%%%%%%%%%%%%%%%%%%%%%%%%%%%%%%%%%%%%%%%%%%%%%%%%%%%%%%%
% assembly of the three separate positive motor velocities (resolution:   %
% 1Byte) and their rotation direction to positive and/or negative         %
% longitudinal, lateral & rotational velocities (in milimeters per        %
% second)                                                                 %
%                                                                         %
% inputs:  direction_motor0_in (rotating direction of motor0              %
%          (129 := counter-clockwise; 128 := clockwise)),                 %
%          velocity_motor0_in (from 0 to 255),                            %
%          direction_motor1_in (rotating direction of motor1              %
%          (0 := counter-clockwise; 1 := clockwise)),                     %
%          velocity_motor1_in (from 0 to 255),                            %
%          direction_motor2_in (rotating direction of motor2              %
%          (0 := counter-clockwise; 1 := clockwise)),                     %
%          velocity_motor2_in (from 0 to 255)                             %
% outputs: v_x_out (longitudinal velocity (in milimeters per second)),    %
%          v_y_out (lateral velocity (in milimeters per second)),         %
%          v_theta_out (rotational velocity (in milimeters per second))   %
%%%%%%%%%%%%%%%%%%%%%%%%%%%%%%%%%%%%%%%%%%%%%%%%%%%%%%%%%%%%%%%%%%%%%%%%%%%
function [v_x_out, v_y_out, v_theta_out] ...
    = fcn(number_of_robot, direction_motor0_in, velocity_motor0_in, direction_motor1_in, ...
          velocity_motor1_in, direction_motor2_in, velocity_motor2_in)
%%%%%%%%%%%%%%%%%%%%%%%%%%%%%%%%%%%%%%%%%%%%%%%%%%%%%%%%%%%%%%%%%
% assembly of absolute motor velocity and rotating direction to %
% longitudinal, lateral & rotational velocity for every motor   %
%%%%%%%%%%%%%%%%%%%%%%%%%%%%%%%%%%%%%%%%%%%%%%%%%%%%%%%%%%%%%%%%%


% the direction bit for the motor 0 of robotino 3 is located at a different position
if number_of_robot == 3
    cmp = 1;
else
    cmp = 129;
end
    

if direction_motor0_in < cmp
    v0 = -velocity_motor0_in;
else
    v0 =  velocity_motor0_in;
end

if direction_motor1_in < 1
    v1 = -velocity_motor1_in;
else
    v1 =  velocity_motor1_in;
end

if direction_motor2_in < 1
    v2 = -velocity_motor2_in;
else
    v2 =  velocity_motor2_in;
end

%%%%%%%%%%%%%%%%%%%%%%%%%%%%%%%%%%%%%%%%%%%%%%%%%%%%%%%%%%%%%%%%%%%%%%%%%
% conversion of the separate motor velocities from a value between -255 %
% and 255 to millimeters                                                %
%%%%%%%%%%%%%%%%%%%%%%%%%%%%%%%%%%%%%%%%%%%%%%%%%%%%%%%%%%%%%%%%%%%%%%%%%
f_rcv = 7.02;
v0    = v0 * f_rcv;
v1    = v1 * f_rcv;
v2    = v2 * f_rcv;

%%%%%%%%%%%%%%%%%%%%%%%%%%%%%%%%%%%%%%%%%%%%%%%%%%%%%%%%%%%%%%%%%%%%
% conversion from three separate motor velocities to longitudinal, %
% lateral & rotational velocity                                    %
%%%%%%%%%%%%%%%%%%%%%%%%%%%%%%%%%%%%%%%%%%%%%%%%%%%%%%%%%%%%%%%%%%%%
v_x_out     = (v2 - v0) / (2 * cosd(30));                         % in mm/s
v_y_out     = (v0 - 2 * v1 + v2) / 3;                             % in mm/s
v_theta_out = (v0 + v1 + v2) / (3 * 135);                        % in rad/s

== stateflow chart Bahnplanung_lauffaehig_auf_Robotino/Bahnplanung/Auftrags_Koordination ==
  settings: updateMethod=DISCRETE  sampleTime=0.005
  state Auftragskoordination
    state WerkstueckAufgenommen
      entry:Werkstueck=1,
      AktuellesZiel=ZielPos;
    state KeinWerkstueckAufgenommen
      entry:Werkstueck=0,
      AktuellesZiel=WerkstueckPos;
    state AufAuftragWarten
      entry:Werkstueck=0,
      AktuellesZiel=100;
    KeinWerkstueckAufgenommen -> WerkstueckAufgenommen : [Werkstueckerkannt==1]
    WerkstueckAufgenommen -> AufAuftragWarten : [Werkstueckerkannt==0]
    AufAuftragWarten -> KeinWerkstueckAufgenommen : [NeuerAuftrag]
    (default) -> AufAuftragWarten
  data: NeuerAuftrag input; WerkstueckPos input; ZielPos input; AktuellesZiel output; Werkstueck output; Werkstueckerkannt input

== matlab function Bahnplanung_lauffaehig_auf_Robotino/Robotino interface/serial communication/stop by bumper ==
  settings: sampleTime=2*dtpc
  data: stop_out output; bumper input; stop_flag_in input; stop_flag_out output
%%%%%%%%%%%%%%%%%%%%%%%%%%%%%%%%%%%%%%%%%%%%%%%%%%%%%%%%%%%%%%%%%%%%%%%%%%%
% Recognition of collisions and creating of variables indicating and      %
% marking a collision                                                     %
%                                                                         %
% inputs: bumper (vector of the three bumper bytes)                       %
%         stop_flag_in (As long as no collision has occured,              %
%                       'stop_flag_in' contains the last bumper vector    %
%                       indicating no collision.                          %
%                       If a collision has occured, 'stop_flag_in'        %
%                       contains the last bumper vector indicating a      %
%                       collision until the simulation stops.)            %
% outputs: stop_out (indicates a collision: 1 = no collision;             %
%                                           0 = collision)                %
%          stop_flag_out (gets the actual bumper vector unless 'bumper'   %
%                         indicates no collision and 'stop_flag_in'       %
%                         indicates a past collision.)                    %
%%%%%%%%%%%%%%%%%%%%%%%%%%%%%%%%%%%%%%%%%%%%%%%%%%%%%%%%%%%%%%%%%%%%%%%%%%%
function [stop_out, stop_flag_out] = fcn(bumper, stop_flag_in)
if max(bumper) == 31       % as soon as the maximum value of the bumper ...
                              % vector indicates 31 a collision is detected
    stop_out = 0;
    stop_flag_out = bumper;
elseif max(stop_flag_in) == 31 % if the maximum value of 'stop_flag_in' ...
                                      % indicates a past collision (31) ...
    stop_out = 0;         % 'stop_out' gets 0 for a further stop of the ...
                                                           % motors and ...
    stop_flag_out = stop_flag_in; % 'stop_flag_out' gets the last bumper...
                                       % vector indicating a past collision
else                                                        % otherwise ...
    stop_out = 1;    % 'stop_out' gets 1 to keep the motors running and ...
    stop_flag_out = bumper; % 'stop_flag_out' gets the actual bumper vector
end

== matlab function Bahnplanung_lauffaehig_auf_Robotino/Robotino interface/distance converter ==
  settings: sampleTime=dtpc/2
  data: dms_in input; dms_out output
%%%%%%%%%%%%%%%%%%%%%%%%%%%%%%%%%%%%%%%%%%%%%%%%%%%%%%%%%%%%%%%%%%%%%%%%%%%
% conversion of the nine distance measuring sensor values (resolution:    %
% 1Byte) to unit milimeters (range: from 40mm to 1500mm) with linear      %
% interpolation                                                           %
%                                                                         %
% input:  vector containing the values of the nine distance measuring     %
%         sensors                                                         %
% output: vector containing the nine values in milimeters                 %
%%%%%%%%%%%%%%%%%%%%%%%%%%%%%%%%%%%%%%%%%%%%%%%%%%%%%%%%%%%%%%%%%%%%%%%%%%%
function dms_out = fcn(dms_in)

y_mm = [40, 45, 50, 60, 75, 100, 125, 150, 175, 200, 250, 300]; % , ...
        %400, 500, 600, 700, 800, 900, 1000, 1100, 1200, 1300, 1500];
    
x_sensor = [255, 249.7733813, 228.6082474, 193.6871795, ...
            152.0044843, 113.7266187, 92.42268041, ...
            76.36407767, 65.19289827, 55.1025641, ...
            43.06299213, 34.97068404]; % , 24.37410072, ...
            % 16.3381295, 11.62589928, 8.661870504, ...
            % 6.316546763, 4.74, 3.65, 2.96, 2.40, ...
            % 2.035971223, 1.539568345];

% x_sensor = round(100 * x_sensor) / 100;

dms_out = interp1(x_sensor, y_mm, dms_in, 'linear');

== matlab function Bahnplanung_lauffaehig_auf_Robotino/Robotino interface/assemble robotino response ==
  data: v_x_in input; robotino_response output; v_y_in input; v_theta_in input; distance_measuring_sensors_in input; bumper_in input; light_barrier_in input; slider_in input
%%%%%%%%%%%%%%%%%%%%%%%%%%%%%%%%%%%%%%%%%%%%%%%%%%%%%%%%%%%%%%%%%%%%%%%%%%%
% Assembly of robot data in a vector of 34 elements.                      %
%                                                                         %
% inputs:   longitudinal, lateral and rotational velocity (in mm/s),      %
%           shaft positions of the three motors (4 elements per motor),   %
%           running times of the three motors (3 elements per motor),     %
%           values of the nine IR-sensors (in mm),                        %
%           bumper collision (1 = no collision;                           %
%                             0 = collision)                              %
% outputs:  vector containing assembled input data                        %
%%%%%%%%%%%%%%%%%%%%%%%%%%%%%%%%%%%%%%%%%%%%%%%%%%%%%%%%%%%%%%%%%%%%%%%%%%%
function robotino_response = fcn(v_x_in, v_y_in, v_theta_in, ...
                                 distance_measuring_sensors_in, ...
                                 bumper_in, light_barrier_in, slider_in)
                                 % motor_positions_in, time_bytes_in, ...)
robotino_response = [light_barrier_in, slider_in, v_x_in, v_y_in, ...
                     v_theta_in, ...%motor_positions_in, time_bytes_in, ...
                     distance_measuring_sensors_in, bumper_in]';

== matlab function Bahnplanung_lauffaehig_auf_Robotino/Robotino interface/light barrier & slider ==
  data: di03_bump_in input; light_barrier output; slider output
function [light_barrier, slider] = fcn(di03_bump_in)
%%%%%%%%%%%%%%%%%%%%%%%%%%%%%%%%%%%%%%%%%%%%%%%%%%%%%%%%%%%%%%%%%%%%%%%%%%%
% di03_bump_in = 0 alternatively 12 ->  no light barrier activation       %
%                                       no slider activation              %
% di03_bump_in = 13                 ->  only light barrier activation     %
% di03_bump_in = 14                 ->  only slider activation            %
% di03_bump_in = 15                 ->  light barrier activation          %
%                                       slider activation                 %
%%%%%%%%%%%%%%%%%%%%%%%%%%%%%%%%%%%%%%%%%%%%%%%%%%%%%%%%%%%%%%%%%%%%%%%%%%%
% function [light_barrier, slider] = fcn(di03_bump_in)
% bin = dec2bin(di03_bump_in);
% if bin(3) == 1
%     light_barrier = 1;
% else
%     light_barrier = 0;
% end
% if bin(4) == 1
%     slider = 1;
% else
%     slider = 0;
% end
if     di03_bump_in == 13
    light_barrier = 1;
    slider        = 0;
elseif di03_bump_in == 14
    light_barrier = 0;
    slider        = 1;
elseif di03_bump_in == 15
    light_barrier = 1;
    slider        = 1;
else
    light_barrier = 0;
    slider        = 0;
end
